simulink model "Building"  (R2016b)
settings: Solver=VariableStepAuto  StartTime=0.0  StopTime=24*3600  FixedStep=10  RelTol=1e-3
model workspace (MAT data in the model file):
  sample_time = 60
libraries: carnot x6
settings Model: Creator=dlindelof  LastModifiedBy=dlindelof

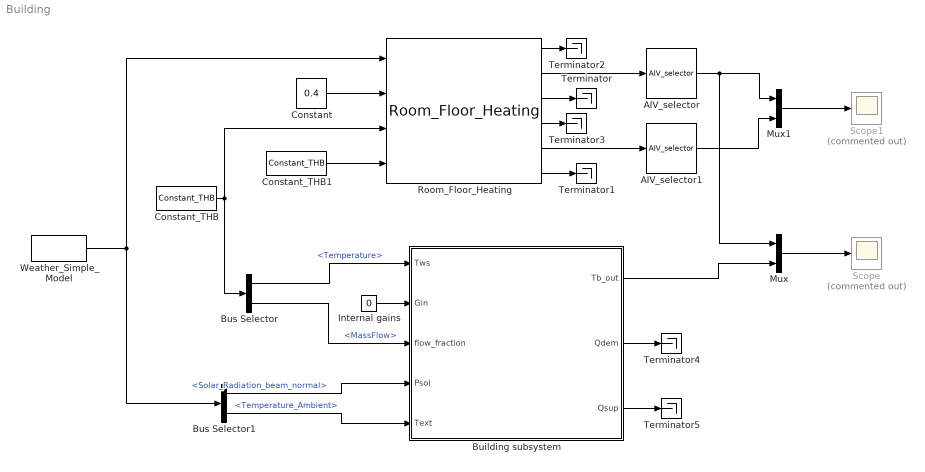
== system Building ==
  AIV_selector : carnot/Outputs/AIV_selector  e1=on  e2=on  e3=on  e4=off  e5=off  e6=off  e7=off  e8=off  e9=off
  AIV_selector1 : carnot/Outputs/AIV_selector  e1=on  e2=on  e3=on  e4=off  e5=off  e6=off  e7=off  e8=off  e9=off
  Building subsystem : Subsystem  TreatAsAtomicUnit=on  SystemSampleTime=sample_time
  Bus Selector : BusSelector  OutputSignals=Temperature,MassFlow
  Bus Selector1 : BusSelector  OutputSignals=Solar_Radiation_beam_normal,Temperature_Ambient
  Constant : Constant  Value=0.4
  Constant_THB : carnot/Source/Simple/Constant_THB  t=30  mdot=600/3600  p=1e5  mID=No Pressure Drop  fluid=Water  mix=0  mix2=0  mix3=0  dia=0.02  hgt=0
  Constant_THB1 : carnot/Source/Simple/Constant_THB  t=30  mdot=600/3600  p=1e5  mID=No Pressure Drop  fluid=Water  mix=0  mix2=0  mix3=0  dia=0.02  hgt=0
  Internal gains : Constant  Value=0
  Mux : Mux  Inputs=2
  Mux1 : Mux  Inputs=2
  Room_Floor_Heating : carnot/Load/Houses/Room_Floor_Heating  t0=20  temp_neighbour=20
  Scope : Scope  Commented=on
  Scope1 : Scope  Commented=on
  Terminator{,1..5} (6 alike) : Terminator
  Weather_Simple_Model : carnot/Weather/Weather_Simple_Model  lat=60  Ibn=900  Idg=100  tamb=5  deltaTsky=-6  rh=50  precip="10e-3/24/3600           % 10 mm in 24 h"  cloud=0.125  p=1013e2  vw=1  wdir=270
  wires:
  Weather_Simple_Model/1 -> Bus Selector1/1, Room_Floor_Heating/1
  Constant/1 -> Room_Floor_Heating/2
  Constant_THB/1 -> Bus Selector/1, Room_Floor_Heating/3
  Constant_THB1/1 -> Room_Floor_Heating/4
  Room_Floor_Heating/2 -> AIV_selector/1
  Room_Floor_Heating/5 -> AIV_selector1/1
  Room_Floor_Heating/3 -> Terminator/1
  Room_Floor_Heating/6 -> Terminator1/1
  Mux1/1 -> Scope1/1
  AIV_selector/1 -> Mux/1, Mux1/1
  AIV_selector1/1 -> Mux1/2
  Room_Floor_Heating/1 -> Terminator2/1
  Room_Floor_Heating/4 -> Terminator3/1
  Bus Selector/1 -> Building subsystem/1(Tws)  "<Temperature>"
  Bus Selector/2 -> Building subsystem/3(flow_fraction)  "<MassFlow>"
  Internal gains/1 -> Building subsystem/2(Gin)
  Bus Selector1/2 -> Building subsystem/5(Text)  "<Temperature_Ambient>"
  Bus Selector1/1 -> Building subsystem/4(Psol)  "<Solar_Radiation_beam_normal>"
  Building subsystem/2(Qdem) -> Terminator4/1
  Building subsystem/3(Qsup) -> Terminator5/1
  Building subsystem/1(Tb_out) -> Mux/2
  Mux/1 -> Scope/1

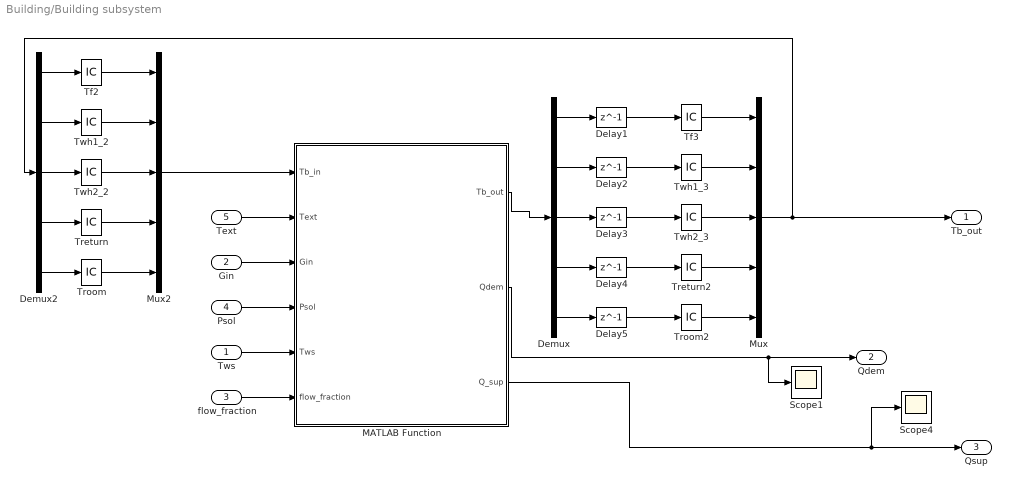
== system Building/Building subsystem ==
  Tws : Inport
  Gin : Inport  Port=2
  flow_fraction : Inport  Port=3
  Psol : Inport  Port=4
  Text : Inport  Port=5
  Delay1 : Delay  DelayLength=1  InitialCondition=0  InputProcessing=Inherited
  Delay2 : Delay  DelayLength=1  InitialCondition=0  InputProcessing=Inherited
  Delay3 : Delay  DelayLength=1  InitialCondition=0
  Delay4 : Delay  DelayLength=1  InitialCondition=0  InputProcessing=Inherited
  Delay5 : Delay  DelayLength=1  InitialCondition=0
  Demux : Demux  Outputs=5
  Demux2 : Demux  Outputs=5
  MATLAB Function : MATLAB Function  TreatAsAtomicUnit=on  mask{sample_time=sample_time}
  Mux : Mux  Inputs=5
  Mux2 : Mux  Inputs=5
  Scope1 : Scope
  Scope4 : Scope
  Tf2 : InitialCondition  Value=22
  Tf3 : InitialCondition  Value=22
  Treturn : InitialCondition  Value=23
  Treturn2 : InitialCondition  Value=23
  Troom : InitialCondition  Value=20
  Troom2 : InitialCondition  Value=20
  Twh1_2 : InitialCondition  Value=25
  Twh1_3 : InitialCondition  Value=25
  Twh2_2 : InitialCondition  Value=24
  Twh2_3 : InitialCondition  Value=24
  Tb_out : Outport
  Qdem : Outport  Port=2
  Qsup : Outport  Port=3
  wires:
  MATLAB Function/1(Tb_out) -> Demux/1
  Demux/2 -> Delay2/1
  Demux/3 -> Delay3/1
  flow_fraction/1 -> MATLAB Function/6(flow_fraction)
  Gin/1 -> MATLAB Function/3(Gin)
  Psol/1 -> MATLAB Function/4(Psol)
  MATLAB Function/2(Qdem) -> Scope1/1, Qdem/1
  Tws/1 -> MATLAB Function/5(Tws)
  Text/1 -> MATLAB Function/2(Text)
  Demux/1 -> Delay1/1
  Demux2/2 -> Twh1_2/1
  Demux2/3 -> Twh2_2/1
  Mux2/1 -> MATLAB Function/1(Tb_in)
  Twh1_2/1 -> Mux2/2
  Twh2_2/1 -> Mux2/3
  Demux2/1 -> Tf2/1
  Tf2/1 -> Mux2/1
  Demux2/4 -> Treturn/1
  Demux2/5 -> Troom/1
  Demux/4 -> Delay4/1
  Demux/5 -> Delay5/1
  Treturn/1 -> Mux2/4
  Troom/1 -> Mux2/5
  Mux/1 -> Demux2/1, Tb_out/1
  Delay2/1 -> Twh1_3/1
  Delay3/1 -> Twh2_3/1
  Delay1/1 -> Tf3/1
  Delay4/1 -> Treturn2/1
  Delay5/1 -> Troom2/1
  Treturn2/1 -> Mux/4
  Twh1_3/1 -> Mux/2
  Troom2/1 -> Mux/5
  Tf3/1 -> Mux/1
  Twh2_3/1 -> Mux/3
  MATLAB Function/3(Q_sup) -> Scope4/1, Qsup/1

== matlab function Building/Building subsystem/MATLAB Function ==
  data: Tb_in input size=[5 1]; Text input; Gin input; Psol input; Tb_out output size=[5 1]; Tws input; flow_fraction input; Qdem output size=1; sample_time parameter; Q_sup output size=1
function [Tb_out, Qdem, Q_sup]  = Simulate_building_dynamics(Tb_in , Text, Gin, Psol, Tws, flow_fraction, sample_time)
%#codegen
% Tf    : Temperature of floor
% Twh1   : water temperature 1 of the heating system pipes
% Twh2   : water temperature 2 of the heating system pipes
% Twr   : Return temperature of the heating system
% Twr   : Return temperature of the heating system
% Tr    : Temperature of the room

% state matrix x = [Tf, Twh1, Twh2, Twr, Tin]';
% input matrix u = [Text, Tws, Gin, Psol]'

[Ab_d, Bb_d,K_fr, K_wf,K_ra, C_wr, mc_f, thermal_capacity_flow] = get_state_input_mat_building(flow_fraction, sample_time);

% F, L,
%Tws = 35;

%Tb_out = Ab_d * Tb_in + Bb_d * [Text; Qsup; Gin; Psol];
Tb_out = Ab_d * Tb_in + Bb_d * [Text; Tws; Gin; Psol];
%Qdem = K_fr * (Tb_out(2)-Tb_out(3));

Qdem = K_ra * (Tb_in(5)-Text)-Psol-Gin;
Q_sup_tot = 4185*flow_fraction*(Tws-Tb_in(4))+((mc_f *(Tb_in(1)-Tb_out(1))) +(C_wr/3)*((Tb_out(2)-Tb_in(2))+(Tb_out(3)-Tb_in(3))+(Tb_out(4)-Tb_in(4))))/sample_time;
% Q_sup1 = 4185*flow_fraction*(Tws-Tb_in(4));
% Q_sup2=(mc_f *(Tb_in(1)-Tb_out(1)))/sample_time;
% Q_sup3=((C_wr/3)*(Tb_out(2)-Tb_in(2)))/sample_time;
% Q_sup4= ((C_wr/3)*(Tb_out(3)-Tb_in(3)))/sample_time;
% Q_sup5= ((C_wr/3)*(Tb_out(4)-Tb_in(4)))/sample_time;
Q_sup = Q_sup_tot; %[Q_sup_tot, Q_sup1, Q_sup2, Q_sup3, Q_sup4, Q_sup5]';


function [Ab_d, Bb_d, K_fr,K_wf,K_ra, C_WH, C_floor, thermal_capacity_flow, Qdot, facHP, nb] = get_state_input_mat_building(floor_heating_flow_fraction, sample_time)

% Create the state matrix and the input matrix for the building system

% state vector for the building
% x_b = [Tf, Twh1, Twh2, Twr, Tin]'

% input vector for the building
% u_b = [Text, Tws, Gin, Psol]';



%[C_return, C_floor, C_room, thermal_capacity_flow, K_wf, K_fr, K_ra, cp_w, Qdot] = get_param_building();
[C_WH, C_floor, C_room, thermal_capacity_flow, K_wf, K_fr, K_ra, cp_w, Qdot] = get_param_building();
%mw_dot = thermal_capacity_flow * floor_heating_flow_fraction;
mw_dot = floor_heating_flow_fraction;

% A = [...
% [ -(K_wf + cp_w*mw_dot)/C_return,          K_wf/C_return,                     0];
% [                   K_wf/C_floor, -(K_fr + K_wf)/C_floor,          K_fr/C_floor];
% [                              0,            K_fr/C_room, -(K_fr + K_ra)/C_room] ...
% ];
% 
% B = [...
% [           0, (cp_w*mw_dot)/C_return,        0,        0];
% [           0,                      0,        0,        0];
% [ K_ra/C_room,                      0, 1/C_room, 1/C_room] ...
% ];

A = [...
[ -(3*K_fr + 3*K_wf)/(3*C_floor),             K_wf/(3*C_floor),             K_wf/(3*C_floor),             K_wf/(3*C_floor),          K_fr/C_floor]
[                      K_wf/C_WH, -(K_wf + 3*cp_w*mw_dot)/C_WH,                            0,                            0,                     0]
[                      K_wf/C_WH,         (3*cp_w*mw_dot)/C_WH, -(K_wf + 3*cp_w*mw_dot)/C_WH,                            0,                     0]
[                      K_wf/C_WH,                            0,         (3*cp_w*mw_dot)/C_WH, -(K_wf + 3*cp_w*mw_dot)/C_WH,                     0]
[                    K_fr/C_room,                            0,                            0,                            0, -(K_fr + K_ra)/C_room]...
];

B = [...
[           0,                    0,        0,        0]
[           0, (3*cp_w*mw_dot)/C_WH,        0,        0]
[           0,                    0,        0,        0]
[           0,                    0,        0,        0]
[ K_ra/C_room,                    0, 1/C_room, 1/C_room]...
];

Ab_d = expm(sample_time*A);
Bb_d = A\(Ab_d-eye(size(A, 1)))*B;


function [C_wr, mc_f, C_r, mdot_d_w, K_wf, K_fr, K_ra, cp_w, Q_D,L_pipes] = get_param_building()
%GET_PARAM_BUILDING returns the parameters of the selected building

cp_w = 4185;        % specific heat of water [J/kgK]
rho_w = 1000;       % density of water [kg/m3]
rho_air = 1.204;    % density of air [kg/m3]
V1 = 0.4;               % Volume of upper layer of storage tank [m3]
V2 = 0.4;               % Volume of middle layer of storage tank [m3]
V3 = 0.4;               % Volume of lower layer of storage tank [m3]
U_wf = 28.2;        %75  % heat transfer coefficient of the distribution pipes [W/m2K] %48.2;
U_fr = 11.7;        % heat transfer coefficient between floor and room [W/m2K]
% \--> Source: On the heat transfer coefficients between heated/cooled radiant floorand room Tomasz Cholewaa
U_ra = 1.19;        % heat transfer coefficient of the wall [W/m2K] 1.19
A_fr = 350;         % floor surface [m2]
A_ra = 600;         % wall surface [m2] 2*2.4H*(6l + 8L)=67.2
d_pipes = 0.033;   % internal diameter of the pipes [m]
d_dz = 0.2;        % space between the pipes [m]
L_pipes = A_fr/d_dz;    % length of the pipe [m]
A_wf = pi*d_pipes*L_pipes; % floor heating pipes surface [m2]
V_w = A_wf*d_pipes/4;      % Volume of water in distribution system [m3]0.228;
V_b = 6300;          % heated volume [m3]
K_wf = U_wf * A_wf; % thermal conductance of the distribution pipes [W/K]
K_fr = U_fr * A_fr; % thermal conductance between floor and room [W/K]
K_ra = U_ra * A_ra; % thermal conductance of the wall [W/K]
tau_r = 10;% 2.4
mc_f = 420e5;       % thermal capacity of the floor [J/K]

C_w = cp_w * rho_w * (V_w);%+V1+V2+V3);   % thermal capacity water [J/K]
%C_r = K_ra * tau_r;         % thermal capacity of the room [J/K]
C_r = V_b * rho_air * 1005 * tau_r; % thermal capacity of the room [J/K]
% Design hydronic system, rules Karlsson_and_Fahlen_2008
Text_D = -10;                   % Design outdoor temperature [K] 
Tin_D = 20;                     % Design outdoor temperature [K] 
Ts_D = 35;                      % Design supply temperature [K]  
Tr_D = 28;                      % Design return temperature [K]
Q_D = K_ra * (Tin_D - Text_D);  % Design heat demand [W]
mdot_d_w = Q_D / ((Ts_D - Tr_D)*cp_w);     % Design mass flow [kg/s]
v = mdot_d_w/(rho_w*(pi*(d_pipes^2)/4));   % Design velocity [m/s]
if v>1.2
    warning('The water velocity in the pipe is too high (noise"s problem are expected. Consider checking the diameter')
end
tau_HP =3*60;                   % Time constant Heat Pump [s]
C_ws = tau_HP * mdot_d_w * cp_w;           % thermal capacity supply water [J/K]
C_wr = C_w; %(C_w - C_ws)*10;        % thermal capacity return water [J/K]
